simulink model "wheels2"  (R2014a)
settings: Solver=ode45  SolverMode=SingleTasking  StartTime=0.0  StopTime=inf  RelTol=1e-3
PreLoadFcn:
  | % Load initialization data
  | 
  | sldemo_absdata;
StopFcn:
  | if exist ('wheels2_output')
  |   wheels2plots;
  | end
undefined symbols (not defined in the file): g, m, mu, Rr, slip, v0
libraries: aerolib6dof2 x1
CloseFcn:
  | % Close the plots that are still open
  | h = findobj(0, 'Name', 'ABS Speeds');
  | if ~isempty(h),
  |   close(h);
  | end;
  | 
  | h = findobj(0, 'Name', 'ABS Slip');
  | if ~isempty(h),
  |   close(h);
  | end;
  | 
  | % Clear initial conditions data to avoid cluttering the workspace
  | 
  | clear g v0 Rr Kf m PBmax TB I slip mu ctrl h;
Description:
  | Modeling an Anti-Lock Braking System (ABS)
  | 
  | *Summary*
  | 
  | This example describes a simple model for an Anti-Lock Braking System
  | (ABS). The model simulates the dynamic behavior of a vehicle
  | under hard braking conditions. The model represents a single wheel, which
  | may be replicated a number of times to create a model for a multi-wheel
  | vehicle.
  | 
  | This model uses the signal logging feature in Simulink(R). You log signals to the
  | MATLAB(R) workspace where you can analyze and view them. You can view
  | the code in sldemo_absbrakeplots.m to see how this is done.
  | 
  | In this model, the wheel speed is calculated in a separate component
  | named sldemo_wheelspeed_absbrake.
  | This component is then referenced using a Model block.  Note that both the
  | top model and the referenced model use a variable step solver, so Simulink
  | will track zero-crossings in the referenced model.
settings Model: FPTRunName=Active  ExtModeTrigMode=oneshot  ExtModeTrigDuration=8  ExtModeArmWhenConnect=off  ExtModeAutoUpdateStatusClock=off  Creator=The MathWorks, Inc.  LastModifiedBy=Abi
settings OptimizationCC: BlockReduction=off  BooleanDataType=off
settings DebuggingCC: SaveWithParameterizedLinksMsg=none  UnderspecifiedInitializationDetection=Classic  SignalResolutionControl=TryResolveAllWithWarning  SolverPrmCheckMsg=none
settings HardwareCC: TargetUnknown=on

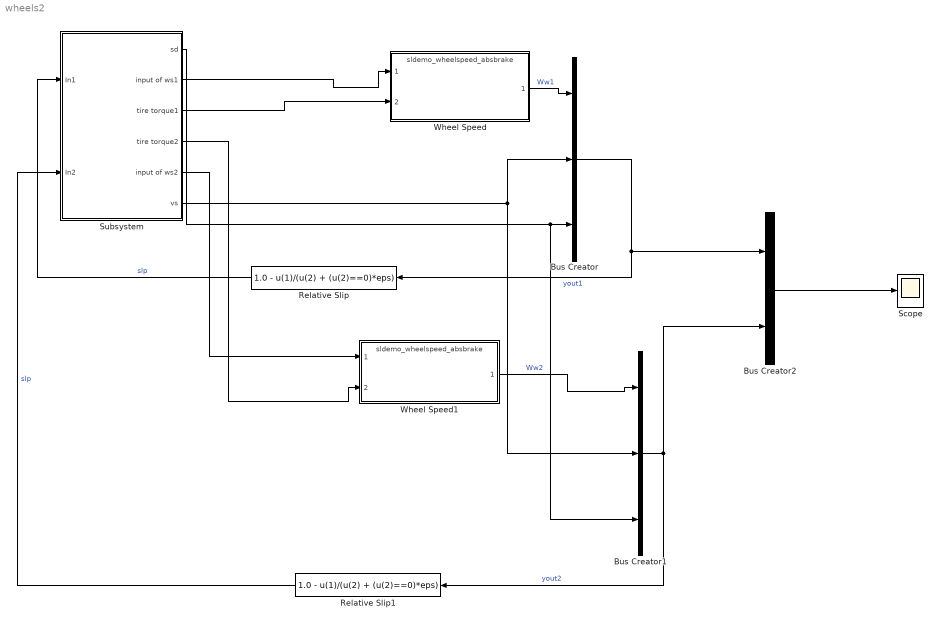
== system wheels2 ==
  Bus Creator2 : BusCreator  Inputs=2
  Bus Creator : BusCreator  Inputs=3
  Bus Creator1 : BusCreator  Inputs=3
  Relative Slip : Fcn  Expr=1.0 - u(1)/(u(2) + (u(2)==0)*eps)
  Relative Slip1 : Fcn  Expr=1.0 - u(1)/(u(2) + (u(2)==0)*eps)
  Scope : Scope
      settings: YMin=0  YMax=6000
  Subsystem : Subsystem
  Wheel Speed : ModelReference  ModelNameDialog=sldemo_wheelspeed_absbrake  SimulationMode=Normal  ModelReferenceVersion=1.65  CopyOfModelName=sldemo_wheelspeed_absbrake  DefaultDataLogging=on
  Wheel Speed1 : ModelReference  ModelNameDialog=sldemo_wheelspeed_absbrake  SimulationMode=Normal  ModelReferenceVersion=1.65  CopyOfModelName=sldemo_wheelspeed_absbrake  DefaultDataLogging=on
  wires:
  Wheel Speed/1 -> Bus Creator/1  "Ww1"
  Relative Slip/1 -> Subsystem/1(In1)  "slp"
  Bus Creator/1 -> Relative Slip/1, Bus Creator2/1  "yout1"
  Wheel Speed1/1 -> Bus Creator1/1  "Ww2"
  Bus Creator1/1 -> Relative Slip1/1, Bus Creator2/2  "yout2"
  Relative Slip1/1 -> Subsystem/2(In2)  "slp"
  Subsystem/1(sd) -> Bus Creator1/3, Bus Creator/3
  Subsystem/2(input of ws1) -> Wheel Speed/1
  Subsystem/3("tire torque1 ") -> Wheel Speed/2
  Subsystem/4(tire torque2) -> Wheel Speed1/2
  Subsystem/6(vs) -> Bus Creator1/2, Bus Creator/2
  Subsystem/5(input of ws2) -> Wheel Speed1/1
  Bus Creator2/1 -> Scope/1

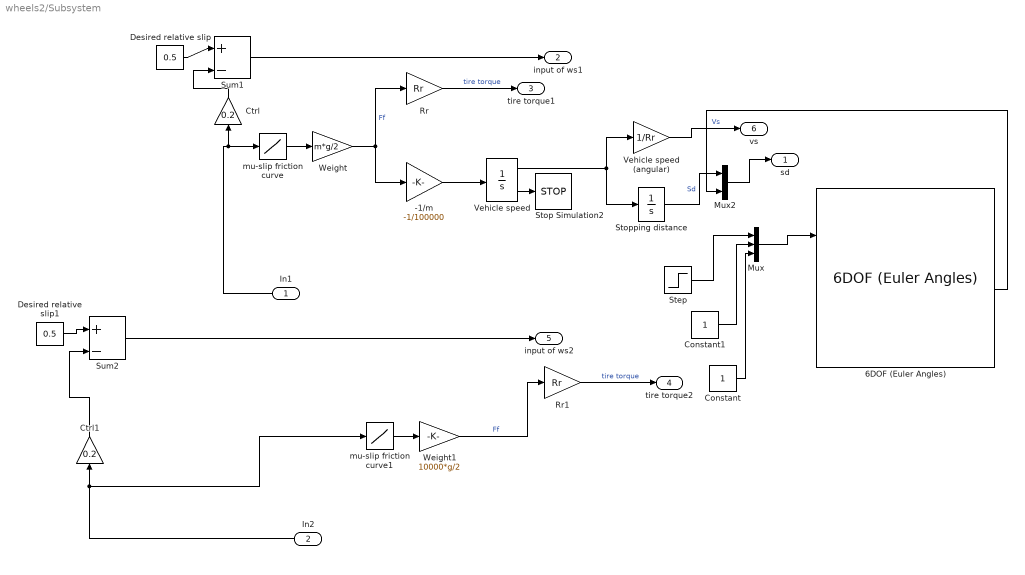
== system wheels2/Subsystem ==
  In1 : Inport
  In2 : Inport  Port=2
  -1/m : Gain  Gain=-1/100000  SaturateOnIntegerOverflow=on  OutDataTypeStr=Inherit: Same as input  ParamDataTypeStr=Inherit: Same as input
  6DOF (Euler Angles) : aerolib6dof2/6DOF (Euler Angles)  units=Metric (MKS)  mtype=Fixed  rep=Euler Angles  xme_0=[0 0 0]  Vm_0=[0 0 0]  eul_0=[0 0 0]  pm_0=[0 0 0]  mass_0=1.0  mass_e=0.5  mass_f=2.0  inertia=eye(3)  inertia_e=eye(3)  inertia_f=2*eye(3)  k_quat=1.0  vre_flag=on
  Constant : Constant
  Constant1 : Constant
  Ctrl : Gain  Gain=0.2  SaturateOnIntegerOverflow=on  OutDataTypeStr=Inherit: Same as input  ParamDataTypeStr=Inherit: Same as input
  Ctrl1 : Gain  Gain=0.2  SaturateOnIntegerOverflow=on  OutDataTypeStr=Inherit: Same as input  ParamDataTypeStr=Inherit: Same as input
  Desired relative slip : Constant  Value=0.5
  Desired relative slip1 : Constant  Value=0.5
  Mux : Mux  Inputs=3
  Mux2 : Mux  Inputs=2
  Rr : Gain  Gain=Rr  SaturateOnIntegerOverflow=on  OutDataTypeStr=Inherit: Same as input  ParamDataTypeStr=Inherit: Same as input
  Rr1 : Gain  Gain=Rr  SaturateOnIntegerOverflow=on  OutDataTypeStr=Inherit: Same as input  ParamDataTypeStr=Inherit: Same as input
  Step : Step  SampleTime=0
  Stop Simulation2 : Stop
  Stopping distance : Integrator  UpperSaturationLimit=1000  LowerSaturationLimit=0
  Sum1 : Sum  Inputs=|+-  SaturateOnIntegerOverflow=on  InputSameDT=on  OutDataTypeStr=Inherit: Same as first input
  Sum2 : Sum  Inputs=|+-  SaturateOnIntegerOverflow=on  InputSameDT=on  OutDataTypeStr=Inherit: Same as first input
  Vehicle speed : Integrator  InitialCondition=v0  LimitOutput=on  UpperSaturationLimit=1000  LowerSaturationLimit=0  ShowSaturationPort=on
  Vehicle speed (angular) : Gain  Gain=1/Rr  SaturateOnIntegerOverflow=on  OutDataTypeStr=Inherit: Same as input  ParamDataTypeStr=Inherit: Same as input
  Weight : Gain  Gain=m*g/2  SaturateOnIntegerOverflow=on  OutDataTypeStr=Inherit: Same as input  ParamDataTypeStr=Inherit: Same as input
  Weight1 : Gain  Gain=10000*g/2  SaturateOnIntegerOverflow=on  OutDataTypeStr=Inherit: Same as input  ParamDataTypeStr=Inherit: Same as input
  mu-slip friction curve : Lookup_n-D  NumberOfTableDimensions=1  BreakpointsForDimension1=slip  Table=mu  SaturateOnIntegerOverflow=on  InputSameDT=on
  mu-slip friction curve1 : Lookup_n-D  NumberOfTableDimensions=1  BreakpointsForDimension1=slip  Table=mu  SaturateOnIntegerOverflow=on  InputSameDT=on
  sd : Outport
  input of ws1 : Outport  Port=2
  "tire torque1 " : Outport  Port=3
  tire torque2 : Outport  Port=4
  input of ws2 : Outport  Port=5
  vs : Outport  Port=6
  wires:
  Weight/1 -> -1/m/1, Rr/1  "Ff"
  Rr/1 -> "tire torque1 "/1  "tire torque"
  Sum1/1 -> input of ws1/1
  mu-slip friction curve/1 -> Weight/1
  -1/m/1 -> Vehicle speed/1
  Desired relative slip/1 -> Sum1/1
  Ctrl/1 -> Sum1/2
  Vehicle speed/2 -> Stop Simulation2/1
  Vehicle speed/1 -> Vehicle speed (angular)/1, Stopping distance/1
  Vehicle speed (angular)/1 -> vs/1  "Vs"
  In1/1 -> mu-slip friction curve/1, Ctrl/1
  Desired relative slip1/1 -> Sum2/1
  Sum2/1 -> input of ws2/1
  Ctrl1/1 -> Sum2/2
  In2/1 -> mu-slip friction curve1/1, Ctrl1/1
  mu-slip friction curve1/1 -> Weight1/1
  Rr1/1 -> tire torque2/1  "tire torque"
  Weight1/1 -> Rr1/1  "Ff"
  Mux/1 -> 6DOF (Euler Angles)/1
  Constant1/1 -> Mux/2
  Constant/1 -> Mux/3
  Step/1 -> Mux/1
  Stopping distance/1 -> Mux2/1  "Sd"
  6DOF (Euler Angles)/5 -> Mux2/2
  Mux2/1 -> sd/1
